simulink model "MMS_ESC_self_driving"  (R2019b)
settings: Solver=VariableStepAuto  StartTime=par.sym.TStart  StopTime=par.sym.TStop  FixedStep=par.sym.max_dt  MaxStep=par.sym.max_dt  RelTol=1e-3
undefined symbols (not defined in the file): B, b, eta_K, k, K_0, lambda_K, m, m1_K0, m2_K0, N_delay, par, Q1_K0, Q2_K0, sigma, T_tran, w_L, w_wav
libraries: simulink x1
settings Model: Creator=Vitù  LastModifiedBy=User
settings SolverCC: AutoInsertRateTranBlk=on
settings DataIOCC: SaveFormat=Array  SaveOutput=off  SignalLogging=off  DSMLogging=off  ReturnWorkspaceOutputs=off  TimeSaveName=TIME  OutputSaveName=Yout  OutputOption=SpecifiedOutputTimes  OutputTimes=[par.sym.TStart:par.sym.Outputdt:par.sym.TStop]
settings OptimizationCC: ExpressionDepthLimit=2147483647  LifeSpan=inf
settings DebuggingCC: UnderspecifiedInitializationDetection=Classic  MergeDetectMultiDrivingBlocksExec=none  SolverPrmCheckMsg=warning  AllowSymbolicDim=off  StateNameClashWarn=warning  SFUnexpectedBacktrackingDiag=warning  SFNoUnconditionalDefaultTransitionDiag=warning  SFExecutionAtInitializationDiag=none  ArithmeticOperatorsInVariantConditions=warning
settings HardwareCC: ProdBitPerPointer=32  ProdBitPerSizeT=32  ProdBitPerPtrDiffT=32  ProdLargestAtomicFloat=None  ProdIntDivRoundTo=Undefined  ProdEndianess=Unspecified  ProdWordSize=32  ProdHWDeviceType=32-bit Generic
settings ModelReferenceCC: PropagateSignalLabelsOutOfModel=off
settings SFSimCC: SimUseLocalCustomCode=off  CustomCodeUndefinedFunction=UseInterfaceOnly
settings RTWCC: RTWUseLocalCustomCode=off
settings CodeAppCC: StateflowObjectComments=on
settings GRTTargetCC: TargetLangStandard=C89/C90 (ANSI)  GeneratePreprocessorConditionals=Disable all
settings ConfigComp: CovMetricSettings=dw  CovHtmlReporting=on  CovSaveCumulativeToWorkspaceVar=on  CovSaveSingleToWorkspaceVar=on  CovExternalEMLEnable=off  CovSFcnEnable=off
settings SimscapeCC: SimscapeNormalizeSystem=off
settings ConfigurationSet: Description=SimMechanics 2G

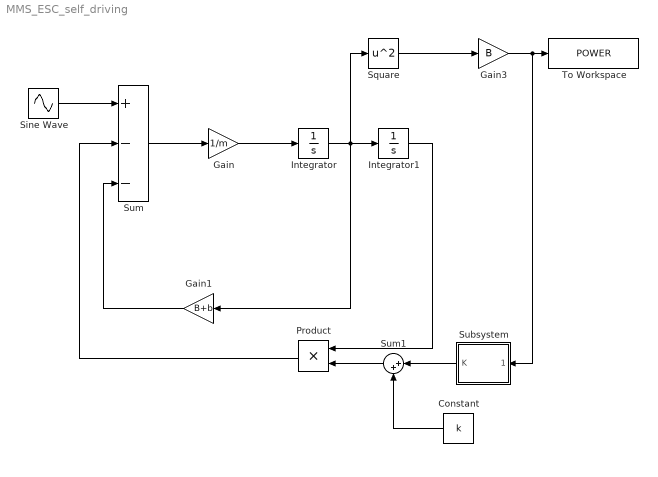
== system MMS_ESC_self_driving ==
  Constant : Constant  Value=k
  Gain : Gain  Gain=1/m
  Gain1 : Gain  Gain=B+b
  Gain3 : Gain  Gain=B
  Integrator : Integrator
  Integrator1 : Integrator
  Product : Product
  Sine Wave : Sin  Amplitude=par.H  Frequency=w_wav  SampleTime=0
  Square : Math  Operator=square  SignedPower=off  SaturateOnIntegerOverflow=on
  Subsystem : Subsystem
  Sum : Sum  Inputs=+--
  Sum1 : Sum  Inputs=|++
  To Workspace : ToWorkspace  VariableName=POWER  SampleTime=-1
  wires:
  Product/1 -> Sum/2
  Gain3/1 -> Subsystem/1(POWER), To Workspace/1
  Integrator/1 -> Square/1, Gain1/1, Integrator1/1
  Gain/1 -> Integrator/1
  Gain1/1 -> Sum/3
  Square/1 -> Gain3/1
  Sum/1 -> Gain/1
  Integrator1/1 -> Product/1
  Sine Wave/1 -> Sum/1
  Subsystem/1(K) -> Sum1/1
  Sum1/1 -> Product/2
  Constant/1 -> Sum1/2

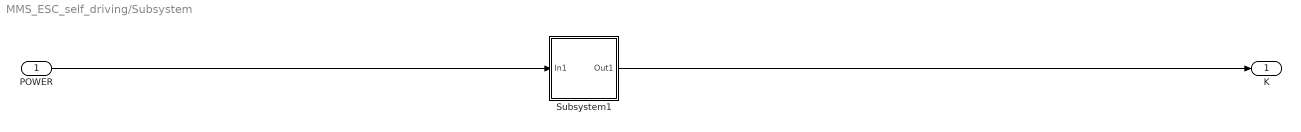
== system MMS_ESC_self_driving/Subsystem ==
  POWER : Inport
  Subsystem1 : Subsystem
  K : Outport
  wires:
  POWER/1 -> Subsystem1/1(In1)
  Subsystem1/1(Out1) -> K/1

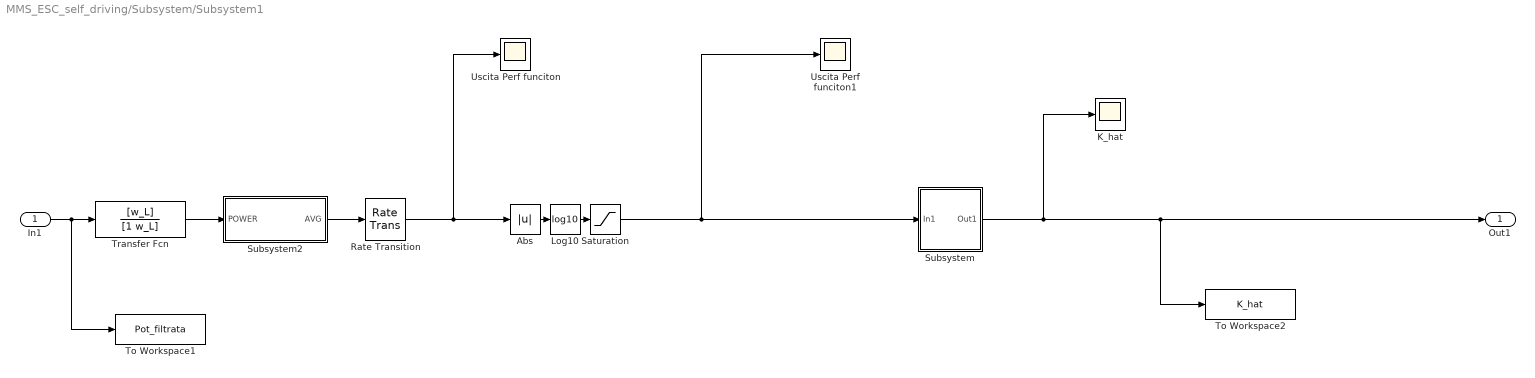
== system MMS_ESC_self_driving/Subsystem/Subsystem1 ==
  In1 : Inport
  Abs : Abs
  K_hat : Scope
  Log10 : Math  Operator=log10  SignedPower=off  SaturateOnIntegerOverflow=on
  Rate Transition : RateTransition
  Saturation : Saturate  UpperLimit=inf  LowerLimit=-20
  Subsystem : Subsystem
  Subsystem2 : Subsystem
  To Workspace1 : ToWorkspace  VariableName=Pot_filtrata  SampleTime=-1
  To Workspace2 : ToWorkspace  VariableName=K_hat  SampleTime=-1
  Transfer Fcn : TransferFcn  Numerator=[w_L]  Denominator=[1 w_L]
  Uscita Perf funciton : Scope
  Uscita Perf funciton1 : Scope
  Out1 : Outport
  wires:
  Rate Transition/1 -> Uscita Perf funciton/1, Abs/1
  Saturation/1 -> Subsystem/1(In1), Uscita Perf funciton1/1
  Abs/1 -> Log10/1
  Subsystem2/1(AVG) -> Rate Transition/1
  Transfer Fcn/1 -> Subsystem2/1(POWER)
  Subsystem/1(Out1) -> To Workspace2/1, Out1/1, K_hat/1
  Log10/1 -> Saturation/1
  In1/1 -> To Workspace1/1, Transfer Fcn/1

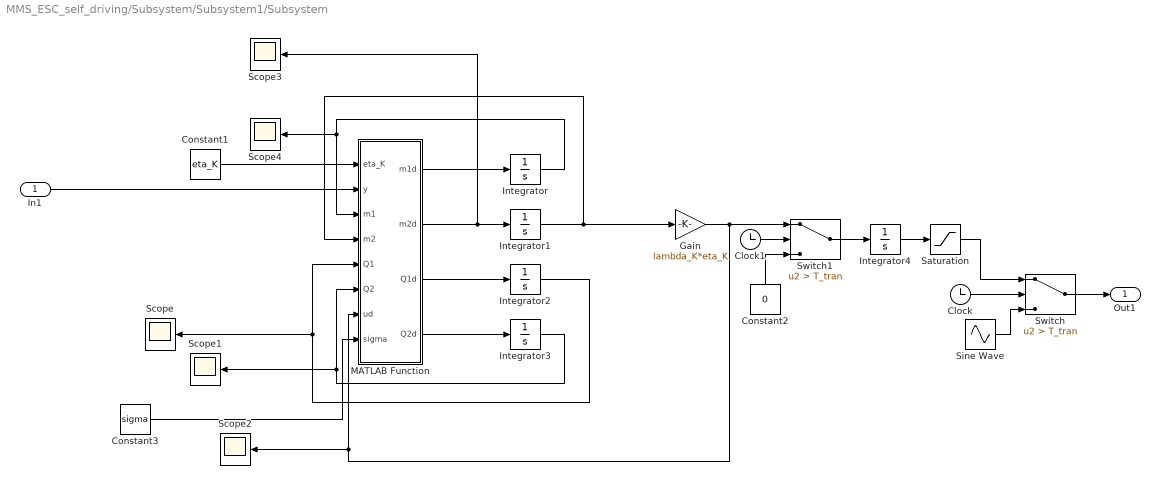
== system MMS_ESC_self_driving/Subsystem/Subsystem1/Subsystem ==
  In1 : Inport
  Clock : Clock
  Clock1 : Clock
  Constant1 : Constant  Value=eta_K
  Constant2 : Constant  Value=0
  Constant3 : Constant  Value=sigma
  Gain : Gain  Gain=lambda_K*eta_K
  Integrator : Integrator  InitialCondition=m1_K0
  Integrator1 : Integrator  InitialCondition=m2_K0
  Integrator2 : Integrator  InitialCondition=Q1_K0
  Integrator3 : Integrator  InitialCondition=Q2_K0
  Integrator4 : Integrator  InitialCondition=K_0
  MATLAB Function : MATLAB Function  TreatAsAtomicUnit=on
  Saturation : Saturate  UpperLimit=inf  LowerLimit=-k
  Scope{,1..4} (5 alike) : Scope
  Sine Wave : Sin  Bias=K_0  SampleTime=0
  Switch : Switch  Criteria=u2 > Threshold  Threshold=T_tran
  Switch1 : Switch  Criteria=u2 > Threshold  Threshold=T_tran
  Out1 : Outport
  wires:
  Sine Wave/1 -> Switch/3
  Gain/1 -> Switch1/1, MATLAB Function/7(ud), Scope2/1
  Constant1/1 -> MATLAB Function/1(eta_K)
  Integrator1/1 -> Gain/1, MATLAB Function/4(m2)
  Integrator3/1 -> MATLAB Function/6(Q2), Scope1/1
  Integrator4/1 -> Saturation/1
  Constant2/1 -> Switch1/3
  Constant3/1 -> MATLAB Function/8(sigma)
  MATLAB Function/1(m1d) -> Integrator/1
  MATLAB Function/2(m2d) -> Scope3/1, Integrator1/1
  MATLAB Function/3(Q1d) -> Integrator2/1
  Integrator/1 -> Scope4/1, MATLAB Function/3(m1)
  MATLAB Function/4(Q2d) -> Integrator3/1
  Clock/1 -> Switch/2
  Integrator2/1 -> MATLAB Function/5(Q1), Scope/1
  Clock1/1 -> Switch1/2
  Switch1/1 -> Integrator4/1
  Switch/1 -> Out1/1
  In1/1 -> MATLAB Function/2(y)
  Saturation/1 -> Switch/1

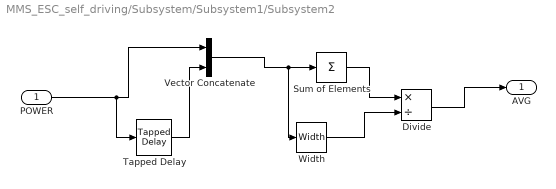
== system MMS_ESC_self_driving/Subsystem/Subsystem1/Subsystem2 ==
  POWER : Inport
  Divide : Product  Inputs=*/
  Sum of Elements : Sum  Inputs=+
  Tapped Delay : simulink/Discrete/Tapped Delay  vinit=0  samptime=-1  NumDelays=N_delay  DelayOrder=Oldest  includeCurrent=off
  Vector Concatenate : Concatenate
  Width : Width
  AVG : Outport
  wires:
  POWER/1 -> Tapped Delay/1, Vector Concatenate/1
  Tapped Delay/1 -> Vector Concatenate/2
  Vector Concatenate/1 -> Width/1, Sum of Elements/1
  Sum of Elements/1 -> Divide/1
  Width/1 -> Divide/2
  Divide/1 -> AVG/1

== matlab function MMS_ESC_self_driving/Subsystem/Subsystem1/Subsystem/MATLAB Function ==
  data: eta_K input; m1d output; y input; m1 input; m2 input; Q1 input; Q2 input; ud input; m2d output; Q1d output; Q2d output; sigma input
function [m1d,m2d,Q1d,Q2d] = SDK(eta_K,y,m1,m2,Q1,Q2,ud,sigma)
m1d = eta_K*(y-m1);
m2d = eta_K*Q1*Q2*(y-m1-Q1*m2)-sigma*eta_K*Q2*m2;
Q1d = -eta_K*Q1 + ud;
Q2d = eta_K*Q2 -eta_K*(Q1*Q2)^2-sigma*eta_K*Q2^2;
